simulink model "robotPrototype"  (R2021a)
settings: Solver=ode15s  StartTime=0.0  StopTime=simTime
model workspace: external: MAT-File (data not in the file)
values from neighbouring files (symbols this model uses):
  controlLim = [0.15 3 3]    [simulinkModelParam.mat]
  controlWeight = [0.75 0.6 0.5]    [simulinkModelParam.mat]
  delta = 0.3    [robotParameters.m]    (also in simulinkModelParam.mat = 0.25)
  deltaPlus = 0.20    (= 0.2)    [robotParameters.m]    (also in simulinkModelParam.mat = 0.15)
  den_CoP = [1 -1.84477840502 0.855986791935]    [simulinkModelParam.mat]
  den_zddot = [1 -1.92894226325 0.931381682127]    [simulinkModelParam.mat]
  f_0 = [1,1; deltaPlus-CoM_0(1), -(delta-deltaPlus+CoM_0(1))]\[m*9.81/2;0]    [robotParameters.m]
  f_sample = 500    [robotParameters.m]    (also in simulinkModelParam.mat = 1000)
  filterCoef = 50    [robotParameters.m]    (also in simulinkModelParam.mat = 1000)
  foot_x = delta    (= 0.3)    [robotParameters.m]    (also in simulinkModelParam.mat = 0.25)
  foot_y = delta/3    (= 0.1)    [robotParameters.m]    (also in simulinkModelParam.mat = 0.0833333333333)
  foot_z = 0.03    [robotParameters.m]    (also in simulinkModelParam.mat = 0.02)
  kd_ank = 0    [robotParameters.m]    (also in simulinkModelParam.mat)
  kd_hip = 250    [robotParameters.m]    (also in simulinkModelParam.mat = 12)
  kd_knee1 = 0.02    [robotParameters.m]    (also in simulinkModelParam.mat = 0)
  kd_knee2 = 500    [robotParameters.m]    (also in simulinkModelParam.mat = 150)
  ki_ank = 1800    [robotParameters.m]    (also in simulinkModelParam.mat = 500)
  ki_hip = 0    [robotParameters.m]    (also in simulinkModelParam.mat)
  ki_knee1 = 0    [robotParameters.m]    (also in simulinkModelParam.mat = 0.5)
  ki_knee2 = 0    [robotParameters.m]    (also in simulinkModelParam.mat)
  kp_ank = 375    [robotParameters.m]    (also in simulinkModelParam.mat = 325)
  kp_hip = 500    [robotParameters.m]    (also in simulinkModelParam.mat = 25)
  kp_knee1 = 8    [robotParameters.m]    (also in simulinkModelParam.mat = 3)
  kp_knee2 = 1000    [robotParameters.m]    (also in simulinkModelParam.mat = 300)
  L = 0.94*2*legLength    (= 0.7896)    [robotParameters.m]    (also in simulinkModelParam.mat = 0.72)
  legLength = param(1)    [forwardKin.m]    (also in robotParameters.m = 0.42; simulinkModelParam.mat = 0.4)
  legWidth = 0.08    [robotParameters.m]    (also in simulinkModelParam.mat = 0.05)
  limbThickness = 0.05    [robotParameters.m]    (also in simulinkModelParam.mat = 0.025)
  m = param(3)    [forwardKin.m]    (also in robotParameters.m = 70; simulinkModelParam.mat = 25)
  modelProperties = [25 0.5781 0.72]    [simulinkModelParam.mat]
  N = length(theta)    [robotParameters.m]
  num_CoP = [0.00280209672777 0.00560419345555 0.00280209672777]    [simulinkModelParam.mat]
  num_zddot = [0.000609854718717 0.00121970943743 0.000609854718717]    [simulinkModelParam.mat]
  p = 28    [simulinkModelParam.mat]
  pushDur = 0.1    [compareReducedOrderModels.m]    (also in simulinkModelParam.mat; startUpBalanceRobot.m)
  pushForce = pushForce - 2*pushStep    (= 0)    [compareReducedOrderModels.m]    (also in startUpBalanceRobot.m = 494)
  pushOnset = 0.2    [compareReducedOrderModels.m]    (also in simulinkModelParam.mat; startUpBalanceRobot.m)
  segmentMass = struct('torso',0.681, 'thigh', 0.2, 'shank', 0.09, 'foot', 0.029)    [robotParameters.m]
  stateLim = [0.15 1.57079632679 0.8 0.55 1.622 0.3]    [simulinkModelParam.mat]
  stateWeight = [3 0.5 0.3 9 0.25 0.09]    [simulinkModelParam.mat]
  support_x = 2.5    [robotParameters.m]    (also in simulinkModelParam.mat)
  support_y = 2.5    [robotParameters.m]    (also in simulinkModelParam.mat)
  support_z = 0.1    [robotParameters.m]    (also in simulinkModelParam.mat)
  torsoCoM = param(2)    [forwardKin.m]    (also in robotParameters.m = 0.235; simulinkModelParam.mat = 0.1875)
  torsoLength = 0.47    [robotParameters.m]    (also in simulinkModelParam.mat = 0.25)
  zmax = (2*legLength)*sin(acos(0.2/(2*legLength)))+ankleOffset    [robotParameters.m]    (also in simulinkModelParam.mat = 0.8)
  zmin = 0.6+ ankleOffset    (= 0.67)    [robotParameters.m]    (also in simulinkModelParam.mat = 0.6)
undefined symbols (not defined in the file or in its folder): controlRateWeight, den_qdot, nlobjLIP, num_qdot, X, Y, Z
libraries: sm_lib x27, nesl_utility x19, pid_lib x16, robotmaniplib x16, simulink_extras x16, mpclib x4, Contact_Forces_Lib x4, simulink x2
(part 3 of 3)

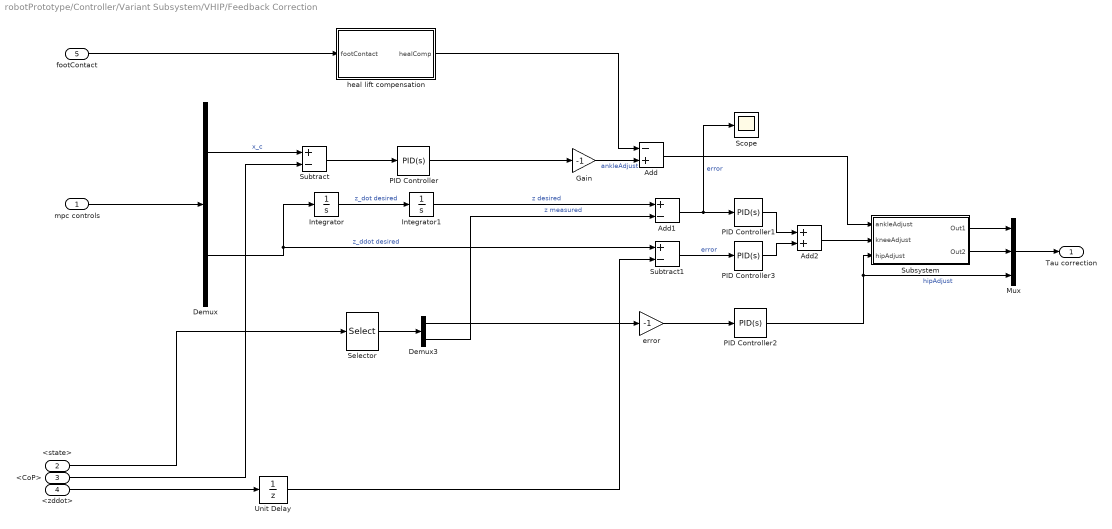
== system robotPrototype/Controller/Variant Subsystem/VHIP/Feedback Correction ==
  mpc controls : Inport
  <state> : Inport  Port=2
  <CoP> : Inport  Port=3
  <zddot> : Inport  Port=4
  footContact : Inport  Port=5
  Add : Sum  Inputs=-+
  Add1 : Sum  Inputs=+-
  Add2 : Sum
  Demux : Demux  Outputs=2
  Demux3 : Demux  Outputs=2
  Gain : Gain  Gain=-1
  Integrator : Integrator
  Integrator1 : Integrator  InitialCondition=L
  Mux : Mux  Inputs=3
  PID Controller : pid_lib/PID Controller  Controller=PID  Form=Parallel  TimeDomain=Continuous-time  UseExternalTs=off  SampleTime=-1  IntegratorMethod=Forward Euler  FilterMethod=Forward Euler  ControllerParametersSource=internal  P=kp_ank+100  I=ki_ank  D=kd_ank  UseFilter=on  N=filterCoef  TunerSelectOption=Transfer Function Based (PID Tuner App)  InitialConditionSource=internal  InitialConditionForIntegrator=0  InitialConditionForFilter=0  DifferentiatorICPrevScaledInput=0  ExternalReset=none  TrackingMode=off  Kt=1  LimitOutput=off  SatLimitsSource=internal  UpperSaturationLimit=inf  LowerSaturationLimit=-inf  LinearizeAsGain=on  AntiWindupMode=none  Kb=1  POutMin=[]  POutMax=[]  IOutMin=[]  IOutMax=[]  DOutMin=[]  DOutMax=[]  NOutMin=[]  NOutMax=[]  SumOutMin=[]  SumOutMax=[]  SaturationOutMin=[]  SaturationOutMax=[]  PParamMin=[]  PParamMax=[]  IParamMin=[]  IParamMax=[]  DParamMin=[]  DParamMax=[]  NParamMin=[]  NParamMax=[]  KbParamMin=[]  KbParamMax=[]  KtParamMin=[]  KtParamMax=[]  KbOutMin=[]  KbOutMax=[]  KtOutMin=[]  KtOutMax=[]  IntegratorOutMin=[]  IntegratorOutMax=[]  FilterOutMin=[]  FilterOutMax=[]  SumI1OutMin=[]  SumI1OutMax=[]  SumI2OutMin=[]  SumI2OutMax=[]  SumI3OutMin=[]  SumI3OutMax=[]  SumI4OutMin=[]  SumI4OutMax=[]  SumDOutMin=[]  SumDOutMax=[]  DifferentiatorOutMin=[]  DifferentiatorOutMax=[]  FilterDiffOutCoefMin=[]  FilterDiffOutCoefMax=[]  ReciprocalOutMin=[]  ReciprocalOutMax=[]  SumDenOutMin=[]  SumDenOutMax=[]  SumNumOutMin=[]  SumNumOutMax=[]  DivideOutMin=[]  DivideOutMax=[]  UdiffTsProdOutMin=[]  UdiffTsProdOutMax=[]  NTsProdOutMin=[]  NTsProdOutMax=[]  UintegralTsProdOutMin=[]  UintegralTsProdOutMax=[]  UngainTsProdOutMin=[]  UngainTsProdOutMax=[]  IntegratorContinuousStateAttributes=''  IntegratorStateMustResolveToSignalObject=off  IntegratorRTWStateStorageClass=Auto  FilterContinuousStateAttributes=''  FilterStateMustResolveToSignalObject=off  FilterRTWStateStorageClass=Auto  ParallelPVariant=InternalParameters  IdealPVariant=Disabled  IVariant=InternalParameters  DVariant=InternalParameters  IntegratorVariant=Continuous  SatVariant=Disabled  AWVariant=Passthrough  PCopyVariant=Disabled  TRVariant=Disabled  FdbkBlocksVariant=Forward  IdealPFdbkVariant=Disabled  SatFdbkVariant=Disabled  DerivativeFilterVariant=ContFilter  NVariant=InternalParameters  NCopyVariant=Disabled  FilterICVariant=InternalICsFilter  IntegratorICVariant=InternalICs  ExternalResetVariant=Disabled  TRSumVariant=Passthrough  SumFdbkVariant=Disabled  SumVariant=Sum_PID  TsampFilterVariant=InternalTs  TsampNgainVariant=Passthrough  TsampIntegralVariant=Passthrough  ExternalSaturationOutDataTypeStr=Inherit: Same as second input
  PID Controller1 : pid_lib/PID Controller  Controller=PID  Form=Parallel  TimeDomain=Continuous-time  UseExternalTs=off  SampleTime=-1  IntegratorMethod=Forward Euler  FilterMethod=Forward Euler  ControllerParametersSource=internal  P=kp_knee2  I=ki_knee2  D=kd_knee2  UseFilter=on  N=filterCoef  TunerSelectOption=Transfer Function Based (PID Tuner App)  InitialConditionSource=internal  InitialConditionForIntegrator=0  InitialConditionForFilter=0  DifferentiatorICPrevScaledInput=0  ExternalReset=none  TrackingMode=off  Kt=1  LimitOutput=off  SatLimitsSource=internal  UpperSaturationLimit=inf  LowerSaturationLimit=-inf  LinearizeAsGain=on  AntiWindupMode=none  Kb=1  POutMin=[]  POutMax=[]  IOutMin=[]  IOutMax=[]  DOutMin=[]  DOutMax=[]  NOutMin=[]  NOutMax=[]  SumOutMin=[]  SumOutMax=[]  SaturationOutMin=[]  SaturationOutMax=[]  PParamMin=[]  PParamMax=[]  IParamMin=[]  IParamMax=[]  DParamMin=[]  DParamMax=[]  NParamMin=[]  NParamMax=[]  KbParamMin=[]  KbParamMax=[]  KtParamMin=[]  KtParamMax=[]  KbOutMin=[]  KbOutMax=[]  KtOutMin=[]  KtOutMax=[]  IntegratorOutMin=[]  IntegratorOutMax=[]  FilterOutMin=[]  FilterOutMax=[]  SumI1OutMin=[]  SumI1OutMax=[]  SumI2OutMin=[]  SumI2OutMax=[]  SumI3OutMin=[]  SumI3OutMax=[]  SumI4OutMin=[]  SumI4OutMax=[]  SumDOutMin=[]  SumDOutMax=[]  DifferentiatorOutMin=[]  DifferentiatorOutMax=[]  FilterDiffOutCoefMin=[]  FilterDiffOutCoefMax=[]  ReciprocalOutMin=[]  ReciprocalOutMax=[]  SumDenOutMin=[]  SumDenOutMax=[]  SumNumOutMin=[]  SumNumOutMax=[]  DivideOutMin=[]  DivideOutMax=[]  UdiffTsProdOutMin=[]  UdiffTsProdOutMax=[]  NTsProdOutMin=[]  NTsProdOutMax=[]  UintegralTsProdOutMin=[]  UintegralTsProdOutMax=[]  UngainTsProdOutMin=[]  UngainTsProdOutMax=[]  IntegratorContinuousStateAttributes=''  IntegratorStateMustResolveToSignalObject=off  IntegratorRTWStateStorageClass=Auto  FilterContinuousStateAttributes=''  FilterStateMustResolveToSignalObject=off  FilterRTWStateStorageClass=Auto  ParallelPVariant=InternalParameters  IdealPVariant=Disabled  IVariant=InternalParameters  DVariant=InternalParameters  IntegratorVariant=Continuous  SatVariant=Disabled  AWVariant=Passthrough  PCopyVariant=Disabled  TRVariant=Disabled  FdbkBlocksVariant=Forward  IdealPFdbkVariant=Disabled  SatFdbkVariant=Disabled  DerivativeFilterVariant=ContFilter  NVariant=InternalParameters  NCopyVariant=Disabled  FilterICVariant=InternalICsFilter  IntegratorICVariant=InternalICs  ExternalResetVariant=Disabled  TRSumVariant=Passthrough  SumFdbkVariant=Disabled  SumVariant=Sum_PID  TsampFilterVariant=InternalTs  TsampNgainVariant=Passthrough  TsampIntegralVariant=Passthrough  ExternalSaturationOutDataTypeStr=Inherit: Same as second input
  PID Controller2 : pid_lib/PID Controller  Controller=PID  Form=Parallel  TimeDomain=Continuous-time  UseExternalTs=off  SampleTime=-1  IntegratorMethod=Forward Euler  FilterMethod=Forward Euler  ControllerParametersSource=internal  P=kp_hip  I=ki_hip  D=kd_hip  UseFilter=on  N=filterCoef  TunerSelectOption=Transfer Function Based (PID Tuner App)  InitialConditionSource=internal  InitialConditionForIntegrator=0  InitialConditionForFilter=0  DifferentiatorICPrevScaledInput=0  ExternalReset=none  TrackingMode=off  Kt=1  LimitOutput=off  SatLimitsSource=internal  UpperSaturationLimit=inf  LowerSaturationLimit=-inf  LinearizeAsGain=on  AntiWindupMode=none  Kb=1  POutMin=[]  POutMax=[]  IOutMin=[]  IOutMax=[]  DOutMin=[]  DOutMax=[]  NOutMin=[]  NOutMax=[]  SumOutMin=[]  SumOutMax=[]  SaturationOutMin=[]  SaturationOutMax=[]  PParamMin=[]  PParamMax=[]  IParamMin=[]  IParamMax=[]  DParamMin=[]  DParamMax=[]  NParamMin=[]  NParamMax=[]  KbParamMin=[]  KbParamMax=[]  KtParamMin=[]  KtParamMax=[]  KbOutMin=[]  KbOutMax=[]  KtOutMin=[]  KtOutMax=[]  IntegratorOutMin=[]  IntegratorOutMax=[]  FilterOutMin=[]  FilterOutMax=[]  SumI1OutMin=[]  SumI1OutMax=[]  SumI2OutMin=[]  SumI2OutMax=[]  SumI3OutMin=[]  SumI3OutMax=[]  SumI4OutMin=[]  SumI4OutMax=[]  SumDOutMin=[]  SumDOutMax=[]  DifferentiatorOutMin=[]  DifferentiatorOutMax=[]  FilterDiffOutCoefMin=[]  FilterDiffOutCoefMax=[]  ReciprocalOutMin=[]  ReciprocalOutMax=[]  SumDenOutMin=[]  SumDenOutMax=[]  SumNumOutMin=[]  SumNumOutMax=[]  DivideOutMin=[]  DivideOutMax=[]  UdiffTsProdOutMin=[]  UdiffTsProdOutMax=[]  NTsProdOutMin=[]  NTsProdOutMax=[]  UintegralTsProdOutMin=[]  UintegralTsProdOutMax=[]  UngainTsProdOutMin=[]  UngainTsProdOutMax=[]  IntegratorContinuousStateAttributes=''  IntegratorStateMustResolveToSignalObject=off  IntegratorRTWStateStorageClass=Auto  FilterContinuousStateAttributes=''  FilterStateMustResolveToSignalObject=off  FilterRTWStateStorageClass=Auto  ParallelPVariant=InternalParameters  IdealPVariant=Disabled  IVariant=InternalParameters  DVariant=InternalParameters  IntegratorVariant=Continuous  SatVariant=Disabled  AWVariant=Passthrough  PCopyVariant=Disabled  TRVariant=Disabled  FdbkBlocksVariant=Forward  IdealPFdbkVariant=Disabled  SatFdbkVariant=Disabled  DerivativeFilterVariant=ContFilter  NVariant=InternalParameters  NCopyVariant=Disabled  FilterICVariant=InternalICsFilter  IntegratorICVariant=InternalICs  ExternalResetVariant=Disabled  TRSumVariant=Passthrough  SumFdbkVariant=Disabled  SumVariant=Sum_PID  TsampFilterVariant=InternalTs  TsampNgainVariant=Passthrough  TsampIntegralVariant=Passthrough  ExternalSaturationOutDataTypeStr=Inherit: Same as second input
  PID Controller3 : pid_lib/PID Controller  Controller=PID  Form=Parallel  TimeDomain=Continuous-time  UseExternalTs=off  SampleTime=-1  IntegratorMethod=Forward Euler  FilterMethod=Forward Euler  ControllerParametersSource=internal  P=kp_knee1  I=ki_knee1  D=kd_knee1  UseFilter=on  N=filterCoef  TunerSelectOption=Frequency Response Based  InitialConditionSource=internal  InitialConditionForIntegrator=0  InitialConditionForFilter=0  DifferentiatorICPrevScaledInput=0  ExternalReset=none  TrackingMode=off  Kt=1  LimitOutput=off  SatLimitsSource=internal  UpperSaturationLimit=inf  LowerSaturationLimit=-inf  LinearizeAsGain=on  AntiWindupMode=none  Kb=1  POutMin=[]  POutMax=[]  IOutMin=[]  IOutMax=[]  DOutMin=[]  DOutMax=[]  NOutMin=[]  NOutMax=[]  SumOutMin=[]  SumOutMax=[]  SaturationOutMin=[]  SaturationOutMax=[]  PParamMin=[]  PParamMax=[]  IParamMin=[]  IParamMax=[]  DParamMin=[]  DParamMax=[]  NParamMin=[]  NParamMax=[]  KbParamMin=[]  KbParamMax=[]  KtParamMin=[]  KtParamMax=[]  KbOutMin=[]  KbOutMax=[]  KtOutMin=[]  KtOutMax=[]  IntegratorOutMin=[]  IntegratorOutMax=[]  FilterOutMin=[]  FilterOutMax=[]  SumI1OutMin=[]  SumI1OutMax=[]  SumI2OutMin=[]  SumI2OutMax=[]  SumI3OutMin=[]  SumI3OutMax=[]  SumI4OutMin=[]  SumI4OutMax=[]  SumDOutMin=[]  SumDOutMax=[]  DifferentiatorOutMin=[]  DifferentiatorOutMax=[]  FilterDiffOutCoefMin=[]  FilterDiffOutCoefMax=[]  ReciprocalOutMin=[]  ReciprocalOutMax=[]  SumDenOutMin=[]  SumDenOutMax=[]  SumNumOutMin=[]  SumNumOutMax=[]  DivideOutMin=[]  DivideOutMax=[]  UdiffTsProdOutMin=[]  UdiffTsProdOutMax=[]  NTsProdOutMin=[]  NTsProdOutMax=[]  UintegralTsProdOutMin=[]  UintegralTsProdOutMax=[]  UngainTsProdOutMin=[]  UngainTsProdOutMax=[]  IntegratorContinuousStateAttributes=''  IntegratorStateMustResolveToSignalObject=off  IntegratorRTWStateStorageClass=Auto  FilterContinuousStateAttributes=''  FilterStateMustResolveToSignalObject=off  FilterRTWStateStorageClass=Auto  ParallelPVariant=InternalParameters  IdealPVariant=Disabled  IVariant=InternalParameters  DVariant=InternalParameters  IntegratorVariant=Continuous  SatVariant=Disabled  AWVariant=Passthrough  PCopyVariant=Disabled  TRVariant=Disabled  FdbkBlocksVariant=Forward  IdealPFdbkVariant=Disabled  SatFdbkVariant=Disabled  DerivativeFilterVariant=ContFilter  NVariant=InternalParameters  NCopyVariant=Disabled  FilterICVariant=InternalICsFilter  IntegratorICVariant=InternalICs  ExternalResetVariant=Disabled  TRSumVariant=Passthrough  SumFdbkVariant=Disabled  SumVariant=Sum_PID  TsampFilterVariant=InternalTs  TsampNgainVariant=Passthrough  TsampIntegralVariant=Passthrough  ExternalSaturationOutDataTypeStr=Inherit: Same as second input
  Scope : Scope
  Selector : Selector  InputPortWidth=6  IndexOptions=Index vector (dialog)  Indices=[2 3]  OutputSizes=1
  Subsystem : Subsystem
  Subtract : Sum  Inputs=+-
  Subtract1 : Sum  Inputs=+-
  Unit Delay : UnitDelay  SampleTime=-1  HasFrameUpgradeWarning=on
  error : Gain  Gain=-1
  heal lift compensation : Subsystem
  Tau correction : Outport
  wires:
  Demux/1 -> Subtract/1  "x_c"
  PID Controller1/1 -> Add2/1
  Add1/1 -> Scope/1, PID Controller1/1  "error"
  mpc controls/1 -> Demux/1
  Demux3/2 -> Add1/2  "z measured"
  Subtract/1 -> PID Controller/1
  Selector/1 -> Demux3/1
  error/1 -> PID Controller2/1
  Demux3/1 -> error/1
  PID Controller2/1 -> Mux/3, Subsystem/3(hipAdjust)  "hipAdjust"
  Demux/2 -> Integrator/1, Subtract1/1  "z_ddot desired"
  Integrator/1 -> Integrator1/1  "z_dot desired"
  <state>/1 -> Selector/1
  Integrator1/1 -> Add1/1  "z desired"
  <CoP>/1 -> Subtract/2
  PID Controller/1 -> Gain/1
  Subtract1/1 -> PID Controller3/1  "error"
  PID Controller3/1 -> Add2/2
  Mux/1 -> Tau correction/1
  <zddot>/1 -> Unit Delay/1
  Unit Delay/1 -> Subtract1/2
  Add2/1 -> Subsystem/2(kneeAdjust)
  Subsystem/1(Out1) -> Mux/1
  Subsystem/2(Out2) -> Mux/2
  footContact/1 -> heal lift compensation/1(footContact)
  Gain/1 -> Add/2  "ankleAdjust"
  heal lift compensation/1(healComp) -> Add/1
  Add/1 -> Subsystem/1(ankleAdjust)

== system robotPrototype/Controller/Variant Subsystem/VHIP/Inverse Dynamics ==
  tau corrective : Inport
  <jointAng> : Inport  Port=2
  Add : Sum  Inputs=+++
  Constant : Constant  Value=zeros(6,4)
  Forward Dynamics : robotmaniplib/Forward Dynamics  RigidBodyTree=robot  SimulateUsing=Code generation
  Gravity Torque : robotmaniplib/Gravity Torque  RigidBodyTree=robot  SimulateUsing=Code generation
  Inverse Dynamics : robotmaniplib/Inverse Dynamics  RigidBodyTree=robot  SimulateUsing=Code generation
      settings: SourceProductBaseCode=RO
  Velocity Product Torque : robotmaniplib/Velocity Product Torque  RigidBodyTree=robot  SimulateUsing=Code generation
      settings: SourceProductBaseCode=RO
  pack joint angles : Subsystem
  tau compesation : Outport
  wires:
  pack joint angles/1(q) -> Velocity Product Torque/1, Gravity Torque/1, Inverse Dynamics/1, Forward Dynamics/1
  <jointAng>/1 -> pack joint angles/1(<jointAng>)
  pack joint angles/2(q_dot) -> Velocity Product Torque/2, Inverse Dynamics/2, Forward Dynamics/2
  Constant/1 -> Forward Dynamics/4, Inverse Dynamics/4
  Forward Dynamics/1 -> Inverse Dynamics/3
  Inverse Dynamics/1 -> tau compesation/1
  Gravity Torque/1 -> Add/1
  Velocity Product Torque/1 -> Add/2
  tau corrective/1 -> Add/3
  Add/1 -> Forward Dynamics/3

== system robotPrototype/Controller/Variant Subsystem/VIPPFW/Inverse Dynamics ==
  tau corrective : Inport
  <jointAng> : Inport  Port=2
  Add : Sum  Inputs=+++
  Constant : Constant  Value=zeros(6,4)
  Forward Dynamics : robotmaniplib/Forward Dynamics  RigidBodyTree=robot  SimulateUsing=Code generation
  Gravity Torque : robotmaniplib/Gravity Torque  RigidBodyTree=robot  SimulateUsing=Code generation
  Inverse Dynamics : robotmaniplib/Inverse Dynamics  RigidBodyTree=robot  SimulateUsing=Code generation
      settings: SourceProductBaseCode=RO
  Velocity Product Torque : robotmaniplib/Velocity Product Torque  RigidBodyTree=robot  SimulateUsing=Code generation
      settings: SourceProductBaseCode=RO
  pack joint angles : Subsystem
  tau compesation : Outport
  wires:
  pack joint angles/1(q) -> Velocity Product Torque/1, Gravity Torque/1, Inverse Dynamics/1, Forward Dynamics/1
  <jointAng>/1 -> pack joint angles/1(<jointAng>)
  pack joint angles/2(q_dot) -> Velocity Product Torque/2, Inverse Dynamics/2, Forward Dynamics/2
  Constant/1 -> Forward Dynamics/4, Inverse Dynamics/4
  Forward Dynamics/1 -> Inverse Dynamics/3
  Inverse Dynamics/1 -> tau compesation/1
  Gravity Torque/1 -> Add/1
  Velocity Product Torque/1 -> Add/2
  tau corrective/1 -> Add/3
  Add/1 -> Forward Dynamics/3

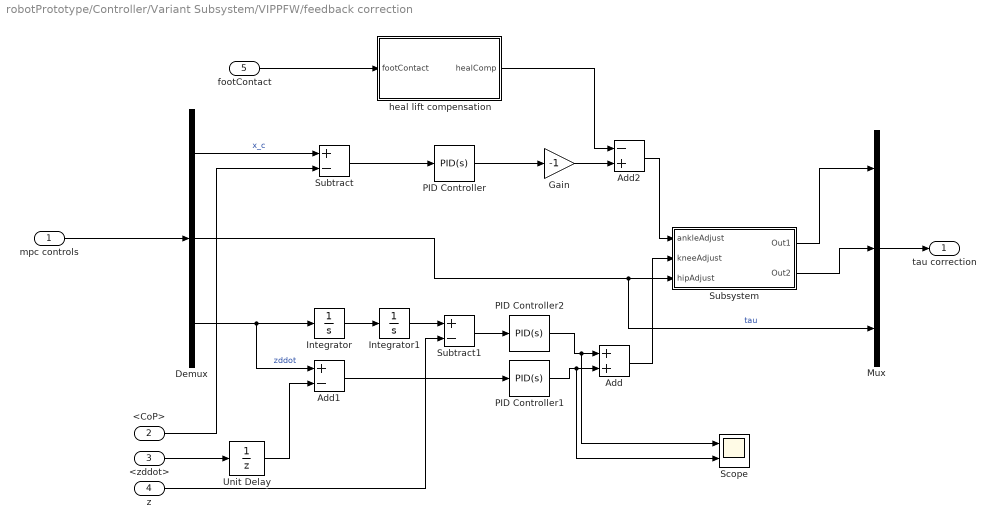
== system robotPrototype/Controller/Variant Subsystem/VIPPFW/feedback correction ==
  mpc controls : Inport
  <CoP> : Inport  Port=2
  <zddot> : Inport  Port=3
  z : Inport  Port=4
  footContact : Inport  Port=5
  Add : Sum
  Add1 : Sum  Inputs=+-
  Add2 : Sum  Inputs=-+
  Demux : Demux  Outputs=3
  Gain : Gain  Gain=-1
  Integrator : Integrator
  Integrator1 : Integrator  InitialCondition=L
  Mux : Mux  Inputs=3
  PID Controller : pid_lib/PID Controller  Controller=PID  Form=Parallel  TimeDomain=Continuous-time  UseExternalTs=off  SampleTime=-1  IntegratorMethod=Forward Euler  FilterMethod=Forward Euler  ControllerParametersSource=internal  P=kp_ank+100  I=ki_ank  D=kd_ank  UseFilter=on  N=filterCoef  TunerSelectOption=Transfer Function Based (PID Tuner App)  InitialConditionSource=internal  InitialConditionForIntegrator=0  InitialConditionForFilter=0  DifferentiatorICPrevScaledInput=0  ExternalReset=none  TrackingMode=off  Kt=1  LimitOutput=off  SatLimitsSource=internal  UpperSaturationLimit=inf  LowerSaturationLimit=-inf  LinearizeAsGain=on  AntiWindupMode=none  Kb=1  POutMin=[]  POutMax=[]  IOutMin=[]  IOutMax=[]  DOutMin=[]  DOutMax=[]  NOutMin=[]  NOutMax=[]  SumOutMin=[]  SumOutMax=[]  SaturationOutMin=[]  SaturationOutMax=[]  PParamMin=[]  PParamMax=[]  IParamMin=[]  IParamMax=[]  DParamMin=[]  DParamMax=[]  NParamMin=[]  NParamMax=[]  KbParamMin=[]  KbParamMax=[]  KtParamMin=[]  KtParamMax=[]  KbOutMin=[]  KbOutMax=[]  KtOutMin=[]  KtOutMax=[]  IntegratorOutMin=[]  IntegratorOutMax=[]  FilterOutMin=[]  FilterOutMax=[]  SumI1OutMin=[]  SumI1OutMax=[]  SumI2OutMin=[]  SumI2OutMax=[]  SumI3OutMin=[]  SumI3OutMax=[]  SumI4OutMin=[]  SumI4OutMax=[]  SumDOutMin=[]  SumDOutMax=[]  DifferentiatorOutMin=[]  DifferentiatorOutMax=[]  FilterDiffOutCoefMin=[]  FilterDiffOutCoefMax=[]  ReciprocalOutMin=[]  ReciprocalOutMax=[]  SumDenOutMin=[]  SumDenOutMax=[]  SumNumOutMin=[]  SumNumOutMax=[]  DivideOutMin=[]  DivideOutMax=[]  UdiffTsProdOutMin=[]  UdiffTsProdOutMax=[]  NTsProdOutMin=[]  NTsProdOutMax=[]  UintegralTsProdOutMin=[]  UintegralTsProdOutMax=[]  UngainTsProdOutMin=[]  UngainTsProdOutMax=[]  IntegratorContinuousStateAttributes=''  IntegratorStateMustResolveToSignalObject=off  IntegratorRTWStateStorageClass=Auto  FilterContinuousStateAttributes=''  FilterStateMustResolveToSignalObject=off  FilterRTWStateStorageClass=Auto  ParallelPVariant=InternalParameters  IdealPVariant=Disabled  IVariant=InternalParameters  DVariant=InternalParameters  IntegratorVariant=Continuous  SatVariant=Disabled  AWVariant=Passthrough  PCopyVariant=Disabled  TRVariant=Disabled  FdbkBlocksVariant=Forward  IdealPFdbkVariant=Disabled  SatFdbkVariant=Disabled  DerivativeFilterVariant=ContFilter  NVariant=InternalParameters  NCopyVariant=Disabled  FilterICVariant=InternalICsFilter  IntegratorICVariant=InternalICs  ExternalResetVariant=Disabled  TRSumVariant=Passthrough  SumFdbkVariant=Disabled  SumVariant=Sum_PID  TsampFilterVariant=InternalTs  TsampNgainVariant=Passthrough  TsampIntegralVariant=Passthrough  ExternalSaturationOutDataTypeStr=Inherit: Same as second input
  PID Controller1 : pid_lib/PID Controller  Controller=PID  Form=Parallel  TimeDomain=Continuous-time  UseExternalTs=off  SampleTime=-1  IntegratorMethod=Forward Euler  FilterMethod=Forward Euler  ControllerParametersSource=internal  P=kp_knee1  I=ki_knee1  D=kd_knee1  UseFilter=on  N=filterCoef  TunerSelectOption=Transfer Function Based (PID Tuner App)  InitialConditionSource=internal  InitialConditionForIntegrator=0  InitialConditionForFilter=0  DifferentiatorICPrevScaledInput=0  ExternalReset=none  TrackingMode=off  Kt=1  LimitOutput=off  SatLimitsSource=internal  UpperSaturationLimit=inf  LowerSaturationLimit=-inf  LinearizeAsGain=on  AntiWindupMode=none  Kb=1  POutMin=[]  POutMax=[]  IOutMin=[]  IOutMax=[]  DOutMin=[]  DOutMax=[]  NOutMin=[]  NOutMax=[]  SumOutMin=[]  SumOutMax=[]  SaturationOutMin=[]  SaturationOutMax=[]  PParamMin=[]  PParamMax=[]  IParamMin=[]  IParamMax=[]  DParamMin=[]  DParamMax=[]  NParamMin=[]  NParamMax=[]  KbParamMin=[]  KbParamMax=[]  KtParamMin=[]  KtParamMax=[]  KbOutMin=[]  KbOutMax=[]  KtOutMin=[]  KtOutMax=[]  IntegratorOutMin=[]  IntegratorOutMax=[]  FilterOutMin=[]  FilterOutMax=[]  SumI1OutMin=[]  SumI1OutMax=[]  SumI2OutMin=[]  SumI2OutMax=[]  SumI3OutMin=[]  SumI3OutMax=[]  SumI4OutMin=[]  SumI4OutMax=[]  SumDOutMin=[]  SumDOutMax=[]  DifferentiatorOutMin=[]  DifferentiatorOutMax=[]  FilterDiffOutCoefMin=[]  FilterDiffOutCoefMax=[]  ReciprocalOutMin=[]  ReciprocalOutMax=[]  SumDenOutMin=[]  SumDenOutMax=[]  SumNumOutMin=[]  SumNumOutMax=[]  DivideOutMin=[]  DivideOutMax=[]  UdiffTsProdOutMin=[]  UdiffTsProdOutMax=[]  NTsProdOutMin=[]  NTsProdOutMax=[]  UintegralTsProdOutMin=[]  UintegralTsProdOutMax=[]  UngainTsProdOutMin=[]  UngainTsProdOutMax=[]  IntegratorContinuousStateAttributes=''  IntegratorStateMustResolveToSignalObject=off  IntegratorRTWStateStorageClass=Auto  FilterContinuousStateAttributes=''  FilterStateMustResolveToSignalObject=off  FilterRTWStateStorageClass=Auto  ParallelPVariant=InternalParameters  IdealPVariant=Disabled  IVariant=InternalParameters  DVariant=InternalParameters  IntegratorVariant=Continuous  SatVariant=Disabled  AWVariant=Passthrough  PCopyVariant=Disabled  TRVariant=Disabled  FdbkBlocksVariant=Forward  IdealPFdbkVariant=Disabled  SatFdbkVariant=Disabled  DerivativeFilterVariant=ContFilter  NVariant=InternalParameters  NCopyVariant=Disabled  FilterICVariant=InternalICsFilter  IntegratorICVariant=InternalICs  ExternalResetVariant=Disabled  TRSumVariant=Passthrough  SumFdbkVariant=Disabled  SumVariant=Sum_PID  TsampFilterVariant=InternalTs  TsampNgainVariant=Passthrough  TsampIntegralVariant=Passthrough  ExternalSaturationOutDataTypeStr=Inherit: Same as second input
  PID Controller2 : pid_lib/PID Controller  Controller=PID  Form=Parallel  TimeDomain=Continuous-time  UseExternalTs=off  SampleTime=-1  IntegratorMethod=Forward Euler  FilterMethod=Forward Euler  ControllerParametersSource=internal  P=kp_knee2  I=ki_knee2  D=kd_knee2  UseFilter=on  N=filterCoef  TunerSelectOption=Transfer Function Based (PID Tuner App)  InitialConditionSource=internal  InitialConditionForIntegrator=0  InitialConditionForFilter=0  DifferentiatorICPrevScaledInput=0  ExternalReset=none  TrackingMode=off  Kt=1  LimitOutput=off  SatLimitsSource=internal  UpperSaturationLimit=inf  LowerSaturationLimit=-inf  LinearizeAsGain=on  AntiWindupMode=none  Kb=1  POutMin=[]  POutMax=[]  IOutMin=[]  IOutMax=[]  DOutMin=[]  DOutMax=[]  NOutMin=[]  NOutMax=[]  SumOutMin=[]  SumOutMax=[]  SaturationOutMin=[]  SaturationOutMax=[]  PParamMin=[]  PParamMax=[]  IParamMin=[]  IParamMax=[]  DParamMin=[]  DParamMax=[]  NParamMin=[]  NParamMax=[]  KbParamMin=[]  KbParamMax=[]  KtParamMin=[]  KtParamMax=[]  KbOutMin=[]  KbOutMax=[]  KtOutMin=[]  KtOutMax=[]  IntegratorOutMin=[]  IntegratorOutMax=[]  FilterOutMin=[]  FilterOutMax=[]  SumI1OutMin=[]  SumI1OutMax=[]  SumI2OutMin=[]  SumI2OutMax=[]  SumI3OutMin=[]  SumI3OutMax=[]  SumI4OutMin=[]  SumI4OutMax=[]  SumDOutMin=[]  SumDOutMax=[]  DifferentiatorOutMin=[]  DifferentiatorOutMax=[]  FilterDiffOutCoefMin=[]  FilterDiffOutCoefMax=[]  ReciprocalOutMin=[]  ReciprocalOutMax=[]  SumDenOutMin=[]  SumDenOutMax=[]  SumNumOutMin=[]  SumNumOutMax=[]  DivideOutMin=[]  DivideOutMax=[]  UdiffTsProdOutMin=[]  UdiffTsProdOutMax=[]  NTsProdOutMin=[]  NTsProdOutMax=[]  UintegralTsProdOutMin=[]  UintegralTsProdOutMax=[]  UngainTsProdOutMin=[]  UngainTsProdOutMax=[]  IntegratorContinuousStateAttributes=''  IntegratorStateMustResolveToSignalObject=off  IntegratorRTWStateStorageClass=Auto  FilterContinuousStateAttributes=''  FilterStateMustResolveToSignalObject=off  FilterRTWStateStorageClass=Auto  ParallelPVariant=InternalParameters  IdealPVariant=Disabled  IVariant=InternalParameters  DVariant=InternalParameters  IntegratorVariant=Continuous  SatVariant=Disabled  AWVariant=Passthrough  PCopyVariant=Disabled  TRVariant=Disabled  FdbkBlocksVariant=Forward  IdealPFdbkVariant=Disabled  SatFdbkVariant=Disabled  DerivativeFilterVariant=ContFilter  NVariant=InternalParameters  NCopyVariant=Disabled  FilterICVariant=InternalICsFilter  IntegratorICVariant=InternalICs  ExternalResetVariant=Disabled  TRSumVariant=Passthrough  SumFdbkVariant=Disabled  SumVariant=Sum_PID  TsampFilterVariant=InternalTs  TsampNgainVariant=Passthrough  TsampIntegralVariant=Passthrough  ExternalSaturationOutDataTypeStr=Inherit: Same as second input
  Scope : Scope  NumInputPorts=2
  Subsystem : Subsystem
  Subtract : Sum  Inputs=+-
  Subtract1 : Sum  Inputs=+-
  Unit Delay : UnitDelay  SampleTime=-1  HasFrameUpgradeWarning=on
  heal lift compensation : Subsystem
  tau correction : Outport
  wires:
  Demux/1 -> Subtract/1  "x_c"
  PID Controller/1 -> Gain/1
  Subtract/1 -> PID Controller/1
  mpc controls/1 -> Demux/1
  Add1/1 -> PID Controller1/1
  Demux/3 -> Add1/1, Integrator/1  "zddot"
  Demux/2 -> Mux/3, Subsystem/3(hipAdjust)  "tau"
  <CoP>/1 -> Subtract/2
  Integrator/1 -> Integrator1/1
  PID Controller2/1 -> Scope/1, Add/1
  PID Controller1/1 -> Scope/2, Add/2
  Integrator1/1 -> Subtract1/1
  z/1 -> Subtract1/2
  Subtract1/1 -> PID Controller2/1
  Mux/1 -> tau correction/1
  <zddot>/1 -> Unit Delay/1
  Unit Delay/1 -> Add1/2
  Subsystem/2(Out2) -> Mux/2
  Add/1 -> Subsystem/2(kneeAdjust)
  Subsystem/1(Out1) -> Mux/1
  Add2/1 -> Subsystem/1(ankleAdjust)
  Gain/1 -> Add2/2
  heal lift compensation/1(healComp) -> Add2/1
  footContact/1 -> heal lift compensation/1(footContact)

== system robotPrototype/Controller/Variant Subsystem/LIP/Feedback Correction/Coupling Correction ==
  ankle : Inport
  nee : Inport  Port=2
  hip : Inport  Port=3
  Add : Sum  Inputs=+++
  Gain1 : Gain  Gain=0.5
  Gain2 : Gain  Gain=.5
  Out1 : Outport
  wires:
  Gain1/1 -> Add/1
  hip/1 -> Gain2/1
  Gain2/1 -> Add/3
  ankle/1 -> Gain1/1
  nee/1 -> Add/2
  Add/1 -> Out1/1

== system robotPrototype/Controller/Variant Subsystem/LIP/Feedback Correction/heal lift compensation ==
  footContact : Inport
  Add : Sum  Inputs=+-
  Bus Selector : BusSelector  OutputSignals=signal5.normalRearTotal
  Constant1 : Constant  Value=2*f_0(1)*0.05
  PID Controller2 : pid_lib/PID Controller  Controller=I  Form=Parallel  TimeDomain=Continuous-time  UseExternalTs=off  SampleTime=-1  IntegratorMethod=Forward Euler  FilterMethod=Forward Euler  ControllerParametersSource=internal  P=1  I=10  D=0  UseFilter=on  N=100  TunerSelectOption=Transfer Function Based (PID Tuner App)  InitialConditionSource=internal  InitialConditionForIntegrator=0  InitialConditionForFilter=0  DifferentiatorICPrevScaledInput=0  ExternalReset=none  TrackingMode=off  Kt=1  LimitOutput=off  SatLimitsSource=internal  UpperSaturationLimit=inf  LowerSaturationLimit=-inf  LinearizeAsGain=on  AntiWindupMode=none  Kb=1  POutMin=[]  POutMax=[]  IOutMin=[]  IOutMax=[]  DOutMin=[]  DOutMax=[]  NOutMin=[]  NOutMax=[]  SumOutMin=[]  SumOutMax=[]  SaturationOutMin=[]  SaturationOutMax=[]  PParamMin=[]  PParamMax=[]  IParamMin=[]  IParamMax=[]  DParamMin=[]  DParamMax=[]  NParamMin=[]  NParamMax=[]  KbParamMin=[]  KbParamMax=[]  KtParamMin=[]  KtParamMax=[]  KbOutMin=[]  KbOutMax=[]  KtOutMin=[]  KtOutMax=[]  IntegratorOutMin=[]  IntegratorOutMax=[]  FilterOutMin=[]  FilterOutMax=[]  SumI1OutMin=[]  SumI1OutMax=[]  SumI2OutMin=[]  SumI2OutMax=[]  SumI3OutMin=[]  SumI3OutMax=[]  SumI4OutMin=[]  SumI4OutMax=[]  SumDOutMin=[]  SumDOutMax=[]  DifferentiatorOutMin=[]  DifferentiatorOutMax=[]  FilterDiffOutCoefMin=[]  FilterDiffOutCoefMax=[]  ReciprocalOutMin=[]  ReciprocalOutMax=[]  SumDenOutMin=[]  SumDenOutMax=[]  SumNumOutMin=[]  SumNumOutMax=[]  DivideOutMin=[]  DivideOutMax=[]  UdiffTsProdOutMin=[]  UdiffTsProdOutMax=[]  NTsProdOutMin=[]  NTsProdOutMax=[]  UintegralTsProdOutMin=[]  UintegralTsProdOutMax=[]  UngainTsProdOutMin=[]  UngainTsProdOutMax=[]  IntegratorContinuousStateAttributes=''  IntegratorStateMustResolveToSignalObject=off  IntegratorRTWStateStorageClass=Auto  FilterContinuousStateAttributes=''  FilterStateMustResolveToSignalObject=off  FilterRTWStateStorageClass=Auto  ParallelPVariant=Disabled  IdealPVariant=Disabled  IVariant=InternalParameters  DVariant=Disabled  IntegratorVariant=Continuous  SatVariant=Disabled  AWVariant=Passthrough  PCopyVariant=Disabled  TRVariant=Disabled  FdbkBlocksVariant=Forward  IdealPFdbkVariant=Disabled  SatFdbkVariant=Disabled  DerivativeFilterVariant=Disabled  NVariant=Disabled  NCopyVariant=Disabled_SignalSpec  FilterICVariant=Disabled  IntegratorICVariant=InternalICs  ExternalResetVariant=Disabled  TRSumVariant=Passthrough  SumFdbkVariant=Disabled  SumVariant=Passthrough_I  TsampFilterVariant=InternalTs  TsampNgainVariant=Passthrough  TsampIntegralVariant=Passthrough  ExternalSaturationOutDataTypeStr=Inherit: Same as second input
  Saturation : Saturate  UpperLimit=0.05*2*f_0(1)  LowerLimit=0
  healComp : Outport
  wires:
  Constant1/1 -> Add/2
  footContact/1 -> Bus Selector/1
  Add/1 -> PID Controller2/1
  Bus Selector/1 -> Saturation/1  "<normalRearTotal>"
  PID Controller2/1 -> healComp/1
  Saturation/1 -> Add/1

== system robotPrototype/Controller/Variant Subsystem/LIP/Inverse Dynamics1/pack joint angles ==
  <jointAng> : Inport
  Demux1 : Demux  Outputs=6
  Mux1 : Mux  Inputs=3
  Mux2 : Mux  Inputs=3
  Transfer Fcn (with initial outputs) : simulink_extras/Additional Linear/Transfer Fcn (with initial outputs)  N=num_qdot  D=den_qdot  Y0=0  U0=0
  Transfer Fcn (with initial outputs)1 : simulink_extras/Additional Linear/Transfer Fcn (with initial outputs)  N=num_qdot  D=den_qdot  Y0=0  U0=0
  Transfer Fcn (with initial outputs)2 : simulink_extras/Additional Linear/Transfer Fcn (with initial outputs)  N=num_qdot  D=den_qdot  Y0=0  U0=0
  q : Outport
  q_dot : Outport  Port=2
  wires:
  Demux1/1 -> Mux1/3
  Demux1/2 -> Mux1/2
  Demux1/3 -> Mux1/1
  Mux1/1 -> q/1
  <jointAng>/1 -> Demux1/1
  Mux2/1 -> q_dot/1
  Transfer Fcn (with initial outputs)/1 -> Mux2/1
  Demux1/6 -> Transfer Fcn (with initial outputs)/1
  Demux1/5 -> Transfer Fcn (with initial outputs)1/1
  Transfer Fcn (with initial outputs)1/1 -> Mux2/2
  Transfer Fcn (with initial outputs)2/1 -> Mux2/3
  Demux1/4 -> Transfer Fcn (with initial outputs)2/1

== system robotPrototype/Controller/Variant Subsystem/LIPPFW/Feedback Compensation/Coupling Correction ==
  In1 : Inport
  In2 : Inport  Port=2
  In3 : Inport  Port=3
  Add : Sum  Inputs=+++
  Gain2 : Gain  Gain=0.5
  Gain3 : Gain  Gain=0.5
  Output : Outport
  wires:
  Gain2/1 -> Add/1
  In2/1 -> Add/2
  Gain3/1 -> Add/3
  In3/1 -> Gain3/1
  In1/1 -> Gain2/1
  Add/1 -> Output/1

== system robotPrototype/Controller/Variant Subsystem/LIPPFW/Feedback Compensation/heal lift compensation ==
  footContact : Inport
  Add : Sum  Inputs=+-
  Bus Selector : BusSelector  OutputSignals=signal5.normalRearTotal
  Constant1 : Constant  Value=2*f_0(1)*0.05
  PID Controller2 : pid_lib/PID Controller  Controller=I  Form=Parallel  TimeDomain=Continuous-time  UseExternalTs=off  SampleTime=-1  IntegratorMethod=Forward Euler  FilterMethod=Forward Euler  ControllerParametersSource=internal  P=1  I=10  D=0  UseFilter=on  N=100  TunerSelectOption=Transfer Function Based (PID Tuner App)  InitialConditionSource=internal  InitialConditionForIntegrator=0  InitialConditionForFilter=0  DifferentiatorICPrevScaledInput=0  ExternalReset=none  TrackingMode=off  Kt=1  LimitOutput=off  SatLimitsSource=internal  UpperSaturationLimit=inf  LowerSaturationLimit=-inf  LinearizeAsGain=on  AntiWindupMode=none  Kb=1  POutMin=[]  POutMax=[]  IOutMin=[]  IOutMax=[]  DOutMin=[]  DOutMax=[]  NOutMin=[]  NOutMax=[]  SumOutMin=[]  SumOutMax=[]  SaturationOutMin=[]  SaturationOutMax=[]  PParamMin=[]  PParamMax=[]  IParamMin=[]  IParamMax=[]  DParamMin=[]  DParamMax=[]  NParamMin=[]  NParamMax=[]  KbParamMin=[]  KbParamMax=[]  KtParamMin=[]  KtParamMax=[]  KbOutMin=[]  KbOutMax=[]  KtOutMin=[]  KtOutMax=[]  IntegratorOutMin=[]  IntegratorOutMax=[]  FilterOutMin=[]  FilterOutMax=[]  SumI1OutMin=[]  SumI1OutMax=[]  SumI2OutMin=[]  SumI2OutMax=[]  SumI3OutMin=[]  SumI3OutMax=[]  SumI4OutMin=[]  SumI4OutMax=[]  SumDOutMin=[]  SumDOutMax=[]  DifferentiatorOutMin=[]  DifferentiatorOutMax=[]  FilterDiffOutCoefMin=[]  FilterDiffOutCoefMax=[]  ReciprocalOutMin=[]  ReciprocalOutMax=[]  SumDenOutMin=[]  SumDenOutMax=[]  SumNumOutMin=[]  SumNumOutMax=[]  DivideOutMin=[]  DivideOutMax=[]  UdiffTsProdOutMin=[]  UdiffTsProdOutMax=[]  NTsProdOutMin=[]  NTsProdOutMax=[]  UintegralTsProdOutMin=[]  UintegralTsProdOutMax=[]  UngainTsProdOutMin=[]  UngainTsProdOutMax=[]  IntegratorContinuousStateAttributes=''  IntegratorStateMustResolveToSignalObject=off  IntegratorRTWStateStorageClass=Auto  FilterContinuousStateAttributes=''  FilterStateMustResolveToSignalObject=off  FilterRTWStateStorageClass=Auto  ParallelPVariant=Disabled  IdealPVariant=Disabled  IVariant=InternalParameters  DVariant=Disabled  IntegratorVariant=Continuous  SatVariant=Disabled  AWVariant=Passthrough  PCopyVariant=Disabled  TRVariant=Disabled  FdbkBlocksVariant=Forward  IdealPFdbkVariant=Disabled  SatFdbkVariant=Disabled  DerivativeFilterVariant=Disabled  NVariant=Disabled  NCopyVariant=Disabled_SignalSpec  FilterICVariant=Disabled  IntegratorICVariant=InternalICs  ExternalResetVariant=Disabled  TRSumVariant=Passthrough  SumFdbkVariant=Disabled  SumVariant=Passthrough_I  TsampFilterVariant=InternalTs  TsampNgainVariant=Passthrough  TsampIntegralVariant=Passthrough  ExternalSaturationOutDataTypeStr=Inherit: Same as second input
  Saturation : Saturate  UpperLimit=0.05*2*f_0(1)  LowerLimit=0
  healComp : Outport
  wires:
  Constant1/1 -> Add/2
  footContact/1 -> Bus Selector/1
  Add/1 -> PID Controller2/1
  Bus Selector/1 -> Saturation/1  "<normalRearTotal>"
  PID Controller2/1 -> healComp/1
  Saturation/1 -> Add/1

== system robotPrototype/Controller/Variant Subsystem/LIPPFW/Inverse Dynamics/pack joint angles ==
  <jointAng> : Inport
  Demux1 : Demux  Outputs=6
  Mux1 : Mux  Inputs=3
  Mux2 : Mux  Inputs=3
  Transfer Fcn (with initial outputs) : simulink_extras/Additional Linear/Transfer Fcn (with initial outputs)  N=num_qdot  D=den_qdot  Y0=0  U0=0
  Transfer Fcn (with initial outputs)1 : simulink_extras/Additional Linear/Transfer Fcn (with initial outputs)  N=num_qdot  D=den_qdot  Y0=0  U0=0
  Transfer Fcn (with initial outputs)2 : simulink_extras/Additional Linear/Transfer Fcn (with initial outputs)  N=num_qdot  D=den_qdot  Y0=0  U0=0
  q : Outport
  q_dot : Outport  Port=2
  wires:
  Demux1/1 -> Mux1/3
  Demux1/2 -> Mux1/2
  Demux1/3 -> Mux1/1
  Mux1/1 -> q/1
  <jointAng>/1 -> Demux1/1
  Mux2/1 -> q_dot/1
  Transfer Fcn (with initial outputs)/1 -> Mux2/1
  Demux1/6 -> Transfer Fcn (with initial outputs)/1
  Demux1/5 -> Transfer Fcn (with initial outputs)1/1
  Transfer Fcn (with initial outputs)1/1 -> Mux2/2
  Transfer Fcn (with initial outputs)2/1 -> Mux2/3
  Demux1/4 -> Transfer Fcn (with initial outputs)2/1

== system robotPrototype/Controller/Variant Subsystem/VHIP/Feedback Correction/Subsystem ==
  ankleAdjust : Inport
  kneeAdjust : Inport  Port=2
  hipAdjust : Inport  Port=3
  Add : Sum  Inputs=+++
  Add3 : Sum
  Gain1 : Gain  Gain=-2
  Gain2 : Gain  Gain=.5
  Gain3 : Gain  Gain=.5
  Out1 : Outport
  Out2 : Outport  Port=2
  wires:
  Add3/1 -> Out1/1
  Gain3/1 -> Add/3
  ankleAdjust/1 -> Add3/1, Gain2/1
  Gain2/1 -> Add/1
  kneeAdjust/1 -> Add/2, Gain1/1
  Add/1 -> Out2/1
  Gain1/1 -> Add3/2
  hipAdjust/1 -> Gain3/1

== system robotPrototype/Controller/Variant Subsystem/VHIP/Feedback Correction/heal lift compensation ==
  footContact : Inport
  Add : Sum  Inputs=+-
  Bus Selector : BusSelector  OutputSignals=signal5.normalRearTotal
  Constant1 : Constant  Value=2*f_0(1)*0.05
  PID Controller2 : pid_lib/PID Controller  Controller=I  Form=Parallel  TimeDomain=Continuous-time  UseExternalTs=off  SampleTime=-1  IntegratorMethod=Forward Euler  FilterMethod=Forward Euler  ControllerParametersSource=internal  P=1  I=10  D=0  UseFilter=on  N=100  TunerSelectOption=Transfer Function Based (PID Tuner App)  InitialConditionSource=internal  InitialConditionForIntegrator=0  InitialConditionForFilter=0  DifferentiatorICPrevScaledInput=0  ExternalReset=none  TrackingMode=off  Kt=1  LimitOutput=off  SatLimitsSource=internal  UpperSaturationLimit=inf  LowerSaturationLimit=-inf  LinearizeAsGain=on  AntiWindupMode=none  Kb=1  POutMin=[]  POutMax=[]  IOutMin=[]  IOutMax=[]  DOutMin=[]  DOutMax=[]  NOutMin=[]  NOutMax=[]  SumOutMin=[]  SumOutMax=[]  SaturationOutMin=[]  SaturationOutMax=[]  PParamMin=[]  PParamMax=[]  IParamMin=[]  IParamMax=[]  DParamMin=[]  DParamMax=[]  NParamMin=[]  NParamMax=[]  KbParamMin=[]  KbParamMax=[]  KtParamMin=[]  KtParamMax=[]  KbOutMin=[]  KbOutMax=[]  KtOutMin=[]  KtOutMax=[]  IntegratorOutMin=[]  IntegratorOutMax=[]  FilterOutMin=[]  FilterOutMax=[]  SumI1OutMin=[]  SumI1OutMax=[]  SumI2OutMin=[]  SumI2OutMax=[]  SumI3OutMin=[]  SumI3OutMax=[]  SumI4OutMin=[]  SumI4OutMax=[]  SumDOutMin=[]  SumDOutMax=[]  DifferentiatorOutMin=[]  DifferentiatorOutMax=[]  FilterDiffOutCoefMin=[]  FilterDiffOutCoefMax=[]  ReciprocalOutMin=[]  ReciprocalOutMax=[]  SumDenOutMin=[]  SumDenOutMax=[]  SumNumOutMin=[]  SumNumOutMax=[]  DivideOutMin=[]  DivideOutMax=[]  UdiffTsProdOutMin=[]  UdiffTsProdOutMax=[]  NTsProdOutMin=[]  NTsProdOutMax=[]  UintegralTsProdOutMin=[]  UintegralTsProdOutMax=[]  UngainTsProdOutMin=[]  UngainTsProdOutMax=[]  IntegratorContinuousStateAttributes=''  IntegratorStateMustResolveToSignalObject=off  IntegratorRTWStateStorageClass=Auto  FilterContinuousStateAttributes=''  FilterStateMustResolveToSignalObject=off  FilterRTWStateStorageClass=Auto  ParallelPVariant=Disabled  IdealPVariant=Disabled  IVariant=InternalParameters  DVariant=Disabled  IntegratorVariant=Continuous  SatVariant=Disabled  AWVariant=Passthrough  PCopyVariant=Disabled  TRVariant=Disabled  FdbkBlocksVariant=Forward  IdealPFdbkVariant=Disabled  SatFdbkVariant=Disabled  DerivativeFilterVariant=Disabled  NVariant=Disabled  NCopyVariant=Disabled_SignalSpec  FilterICVariant=Disabled  IntegratorICVariant=InternalICs  ExternalResetVariant=Disabled  TRSumVariant=Passthrough  SumFdbkVariant=Disabled  SumVariant=Passthrough_I  TsampFilterVariant=InternalTs  TsampNgainVariant=Passthrough  TsampIntegralVariant=Passthrough  ExternalSaturationOutDataTypeStr=Inherit: Same as second input
  Saturation : Saturate  UpperLimit=0.05*2*f_0(1)  LowerLimit=0
  healComp : Outport
  wires:
  Constant1/1 -> Add/2
  footContact/1 -> Bus Selector/1
  Add/1 -> PID Controller2/1
  Bus Selector/1 -> Saturation/1  "<normalRearTotal>"
  PID Controller2/1 -> healComp/1
  Saturation/1 -> Add/1

== system robotPrototype/Controller/Variant Subsystem/VHIP/Inverse Dynamics/pack joint angles ==
  <jointAng> : Inport
  Demux1 : Demux  Outputs=6
  Mux1 : Mux  Inputs=3
  Mux2 : Mux  Inputs=3
  Transfer Fcn (with initial outputs) : simulink_extras/Additional Linear/Transfer Fcn (with initial outputs)  N=num_qdot  D=den_qdot  Y0=0  U0=0
  Transfer Fcn (with initial outputs)1 : simulink_extras/Additional Linear/Transfer Fcn (with initial outputs)  N=num_qdot  D=den_qdot  Y0=0  U0=0
  Transfer Fcn (with initial outputs)2 : simulink_extras/Additional Linear/Transfer Fcn (with initial outputs)  N=num_qdot  D=den_qdot  Y0=0  U0=0
  q : Outport
  q_dot : Outport  Port=2
  wires:
  Demux1/1 -> Mux1/3
  Demux1/2 -> Mux1/2
  Demux1/3 -> Mux1/1
  Mux1/1 -> q/1
  <jointAng>/1 -> Demux1/1
  Mux2/1 -> q_dot/1
  Transfer Fcn (with initial outputs)/1 -> Mux2/1
  Demux1/6 -> Transfer Fcn (with initial outputs)/1
  Demux1/5 -> Transfer Fcn (with initial outputs)1/1
  Transfer Fcn (with initial outputs)1/1 -> Mux2/2
  Transfer Fcn (with initial outputs)2/1 -> Mux2/3
  Demux1/4 -> Transfer Fcn (with initial outputs)2/1

== system robotPrototype/Controller/Variant Subsystem/VIPPFW/Inverse Dynamics/pack joint angles ==
  <jointAng> : Inport
  Demux1 : Demux  Outputs=6
  Mux1 : Mux  Inputs=3
  Mux2 : Mux  Inputs=3
  Transfer Fcn (with initial outputs) : simulink_extras/Additional Linear/Transfer Fcn (with initial outputs)  N=num_qdot  D=den_qdot  Y0=0  U0=0
  Transfer Fcn (with initial outputs)1 : simulink_extras/Additional Linear/Transfer Fcn (with initial outputs)  N=num_qdot  D=den_qdot  Y0=0  U0=0
  Transfer Fcn (with initial outputs)2 : simulink_extras/Additional Linear/Transfer Fcn (with initial outputs)  N=num_qdot  D=den_qdot  Y0=0  U0=0
  q : Outport
  q_dot : Outport  Port=2
  wires:
  Demux1/1 -> Mux1/3
  Demux1/2 -> Mux1/2
  Demux1/3 -> Mux1/1
  Mux1/1 -> q/1
  <jointAng>/1 -> Demux1/1
  Mux2/1 -> q_dot/1
  Transfer Fcn (with initial outputs)/1 -> Mux2/1
  Demux1/6 -> Transfer Fcn (with initial outputs)/1
  Demux1/5 -> Transfer Fcn (with initial outputs)1/1
  Transfer Fcn (with initial outputs)1/1 -> Mux2/2
  Transfer Fcn (with initial outputs)2/1 -> Mux2/3
  Demux1/4 -> Transfer Fcn (with initial outputs)2/1

== system robotPrototype/Controller/Variant Subsystem/VIPPFW/feedback correction/Subsystem ==
  ankleAdjust : Inport
  kneeAdjust : Inport  Port=2
  hipAdjust : Inport  Port=3
  Add : Sum  Inputs=+++
  Add3 : Sum
  Gain1 : Gain  Gain=-2
  Gain2 : Gain  Gain=.5
  Gain3 : Gain  Gain=.5
  Out1 : Outport
  Out2 : Outport  Port=2
  wires:
  Add3/1 -> Out1/1
  Gain3/1 -> Add/3
  ankleAdjust/1 -> Add3/1, Gain2/1
  Gain2/1 -> Add/1
  kneeAdjust/1 -> Add/2, Gain1/1
  Add/1 -> Out2/1
  Gain1/1 -> Add3/2
  hipAdjust/1 -> Gain3/1

== system robotPrototype/Controller/Variant Subsystem/VIPPFW/feedback correction/heal lift compensation ==
  footContact : Inport
  Add : Sum  Inputs=+-
  Bus Selector : BusSelector  OutputSignals=signal5.normalRearTotal
  Constant1 : Constant  Value=2*f_0(1)*0.05
  PID Controller2 : pid_lib/PID Controller  Controller=I  Form=Parallel  TimeDomain=Continuous-time  UseExternalTs=off  SampleTime=-1  IntegratorMethod=Forward Euler  FilterMethod=Forward Euler  ControllerParametersSource=internal  P=1  I=10  D=0  UseFilter=on  N=100  TunerSelectOption=Transfer Function Based (PID Tuner App)  InitialConditionSource=internal  InitialConditionForIntegrator=0  InitialConditionForFilter=0  DifferentiatorICPrevScaledInput=0  ExternalReset=none  TrackingMode=off  Kt=1  LimitOutput=off  SatLimitsSource=internal  UpperSaturationLimit=inf  LowerSaturationLimit=-inf  LinearizeAsGain=on  AntiWindupMode=none  Kb=1  POutMin=[]  POutMax=[]  IOutMin=[]  IOutMax=[]  DOutMin=[]  DOutMax=[]  NOutMin=[]  NOutMax=[]  SumOutMin=[]  SumOutMax=[]  SaturationOutMin=[]  SaturationOutMax=[]  PParamMin=[]  PParamMax=[]  IParamMin=[]  IParamMax=[]  DParamMin=[]  DParamMax=[]  NParamMin=[]  NParamMax=[]  KbParamMin=[]  KbParamMax=[]  KtParamMin=[]  KtParamMax=[]  KbOutMin=[]  KbOutMax=[]  KtOutMin=[]  KtOutMax=[]  IntegratorOutMin=[]  IntegratorOutMax=[]  FilterOutMin=[]  FilterOutMax=[]  SumI1OutMin=[]  SumI1OutMax=[]  SumI2OutMin=[]  SumI2OutMax=[]  SumI3OutMin=[]  SumI3OutMax=[]  SumI4OutMin=[]  SumI4OutMax=[]  SumDOutMin=[]  SumDOutMax=[]  DifferentiatorOutMin=[]  DifferentiatorOutMax=[]  FilterDiffOutCoefMin=[]  FilterDiffOutCoefMax=[]  ReciprocalOutMin=[]  ReciprocalOutMax=[]  SumDenOutMin=[]  SumDenOutMax=[]  SumNumOutMin=[]  SumNumOutMax=[]  DivideOutMin=[]  DivideOutMax=[]  UdiffTsProdOutMin=[]  UdiffTsProdOutMax=[]  NTsProdOutMin=[]  NTsProdOutMax=[]  UintegralTsProdOutMin=[]  UintegralTsProdOutMax=[]  UngainTsProdOutMin=[]  UngainTsProdOutMax=[]  IntegratorContinuousStateAttributes=''  IntegratorStateMustResolveToSignalObject=off  IntegratorRTWStateStorageClass=Auto  FilterContinuousStateAttributes=''  FilterStateMustResolveToSignalObject=off  FilterRTWStateStorageClass=Auto  ParallelPVariant=Disabled  IdealPVariant=Disabled  IVariant=InternalParameters  DVariant=Disabled  IntegratorVariant=Continuous  SatVariant=Disabled  AWVariant=Passthrough  PCopyVariant=Disabled  TRVariant=Disabled  FdbkBlocksVariant=Forward  IdealPFdbkVariant=Disabled  SatFdbkVariant=Disabled  DerivativeFilterVariant=Disabled  NVariant=Disabled  NCopyVariant=Disabled_SignalSpec  FilterICVariant=Disabled  IntegratorICVariant=InternalICs  ExternalResetVariant=Disabled  TRSumVariant=Passthrough  SumFdbkVariant=Disabled  SumVariant=Passthrough_I  TsampFilterVariant=InternalTs  TsampNgainVariant=Passthrough  TsampIntegralVariant=Passthrough  ExternalSaturationOutDataTypeStr=Inherit: Same as second input
  Saturation : Saturate  UpperLimit=0.05*2*f_0(1)  LowerLimit=0
  healComp : Outport
  wires:
  Constant1/1 -> Add/2
  footContact/1 -> Bus Selector/1
  Add/1 -> PID Controller2/1
  Bus Selector/1 -> Saturation/1  "<normalRearTotal>"
  PID Controller2/1 -> healComp/1
  Saturation/1 -> Add/1

== matlab function robotPrototype/Robot/Measures State/MATLAB Function ==
  settings: updateMethod=DISCRETE
  data: q input; X_com output; X_hip input; phi input; param input; X_knee output; X_ank output
function [X_com,X_knee,X_ank]  = fcn(q,X_hip,phi,param)
% call forward kin


[X_com,X_knee,X_ank] = forwardKin(q,X_hip,-phi,param);
